simulink model "servo1"  (R2015a)
settings: Solver=ode45  StartTime=0.0  StopTime=10.0  RelTol=1e-3
values from neighbouring files (symbols this model uses):
  A = [0 1 0 0 ... (first row only)    [following.m]    (also in hoge.m = [0 1; servo.m)
  B = [0 2 0 0]'    [following.m]    (also in hoge.m = [0 1]'; servo.m)
  c = [0 0 1 0]    [following.m]    (also in servo.m)
  C = eye(4)    [following.m]    (also in hoge.m = [1 0]; servo.m)
  D = zeros(4,1)    [following.m]    (also in hoge.m = 0; servo.m)
  G = Ke(5)    [servo.m]
  K = -acker(A,B,p)    [following.m]    (also in servo.m = Ke(1:4))
  x0 = zeros(4,1)    [following.m]    (also in hoge.m = [1 0]'; servo.m)
settings Model: Creator=shohei  LastModifiedBy=shohei

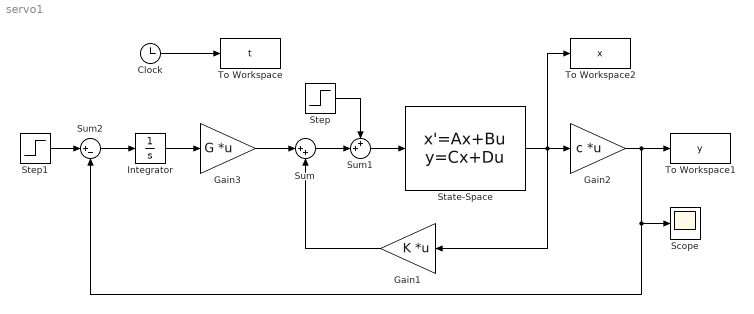
== system servo1 ==
  Clock : Clock
  Gain1 : Gain  Gain=K  Multiplication=Matrix(K*u)
  Gain2 : Gain  Gain=c  Multiplication=Matrix(K*u)
  Gain3 : Gain  Gain=G  Multiplication=Matrix(K*u)
  Integrator : Integrator
  Scope : Scope
  State-Space : StateSpace  A=A  B=B  C=C  D=D  X0=x0
  Step : Step  Time=5  SampleTime=0
  Step1 : Step  Time=0  SampleTime=0
  Sum : Sum  Inputs=|++
  Sum1 : Sum  Inputs=++|
  Sum2 : Sum  Inputs=|+-
  To Workspace : ToWorkspace  VariableName=t  SampleTime=-1
  To Workspace1 : ToWorkspace  VariableName=y  SampleTime=-1
  To Workspace2 : ToWorkspace  VariableName=x  SampleTime=-1
  wires:
  Sum/1 -> Sum1/2
  Step/1 -> Sum1/1
  Sum1/1 -> State-Space/1
  Gain1/1 -> Sum/2
  State-Space/1 -> Gain1/1, To Workspace2/1, Gain2/1
  Gain2/1 -> Sum2/2, Scope/1, To Workspace1/1
  Clock/1 -> To Workspace/1
  Sum2/1 -> Integrator/1
  Step1/1 -> Sum2/1
  Integrator/1 -> Gain3/1
  Gain3/1 -> Sum/1
